simulink model "Communication6_2018a"  (R2018a)
settings: Solver=VariableStepAuto  StartTime=0.0  StopTime=0.6  RelTol=1e-3
settings Model: Creator=86188  LastModifiedBy=bzhan

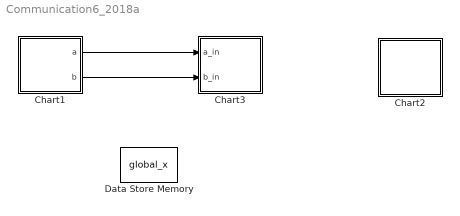
== system Communication6_2018a ==
  Chart1 : Stateflow chart  TreatAsAtomicUnit=on
  Chart2 : Stateflow chart  TreatAsAtomicUnit=on
  Chart3 : Stateflow chart  TreatAsAtomicUnit=on
  Data Store Memory : DataStoreMemory  DataStoreName=global_x  ReadBeforeWriteMsg=warning  WriteAfterWriteMsg=warning  WriteAfterReadMsg=warning  ShowAdditionalParam=off  OutDataTypeStr=int32
  wires:
  Chart1/2(b) -> Chart3/2(b_in)
  Chart1/1(a) -> Chart3/1(a_in)

== stateflow chart Communication6_2018a/Chart3 ==
  settings: updateMethod=DISCRETE  sampleTime=0.1
  state A1
    en: g("en_A1")
    du: f()
  (default) -> A1
  data: s function_input; a_in input; b_in input; global_x data_store_memory
  function f:
    | function f
    |   fprintf("%.0f %.0f\n", a_in, b_in);
  function g(s):
    | function g(s)
    |   fprintf(s+"\n");

== stateflow chart Communication6_2018a/Chart2 ==
  settings: updateMethod=DISCRETE  sampleTime=0.1
  state C
    en: g("en_C")
    du: f()
  (default) -> C
  data: s function_input; global_x data_store_memory
  function f:
    | function f
    |   fprintf("%d\n", global_x);
  function g(s):
    | function g(s)
    |   fprintf(s+"\n");

== stateflow chart Communication6_2018a/Chart1 ==
  settings: updateMethod=DISCRETE  sampleTime=0.1
  state A
    en:
    f("en_A")
  state B
    en:
    f("en_B")
  (default) -> A : {a=1;b=1;}
  A -> B : {a=a+1; global_x=global_x+1;}
  B -> A : {b=b+1;}
  data: s function_input; a output; b output; global_x data_store_memory
  function f(s):
    | function f(s)
    |   fprintf(s+"\n");
